simulink model "unitree_a1_bounding"  (R2022b)
settings: Solver=VariableStepAuto  StartTime=0.0  StopTime=10.0  RelTol=1e-3
values from neighbouring files (symbols this model uses):
  m = 12    [mpc.m]    (also in mpc_soln.m; qp_soln.m)
  N = 50    [mpc.m]    (also in mpc_caller.m = params.N; qp_caller.m = params.N)
  X = [p; reshape(R, [9 1]); v; R'*w]    [mpc_caller.m]    (also in qp_caller.m)
undefined symbols (not defined in the file or in its folder): Y, Z
libraries: sm_lib x214, nesl_utility x117, simulink x3
(part 4 of 5)

== system unitree_a1_bounding/Subsystem4 ==
  PS-Simulink Converter : nesl_utility/PS-Simulink Converter  PhysicalDomain=network_engine_domain  SubClassName=ps_output  LeftPortType=input  RightPortType=output  PseudoPeriodic=off  Frequencies=[]  VectorFormat=inherit  Unit=inherit  AffineConversion=off
  PS-Simulink Converter1 : nesl_utility/PS-Simulink Converter  PhysicalDomain=network_engine_domain  SubClassName=ps_output  LeftPortType=input  RightPortType=output  PseudoPeriodic=off  Frequencies=[]  VectorFormat=inherit  Unit=inherit  AffineConversion=off
  PS-Simulink Converter2 : nesl_utility/PS-Simulink Converter  PhysicalDomain=network_engine_domain  SubClassName=ps_output  LeftPortType=input  RightPortType=output  PseudoPeriodic=off  Frequencies=[]  VectorFormat=inherit  Unit=inherit  AffineConversion=off
  1 : PMIOPort  Side=Left
  2 : PMIOPort  Port=2  Side=Left
  3 : PMIOPort  Port=3  Side=Left
  q : Outport
  w : Outport  Port=2
  t : Outport  Port=3
  wires:
  PS-Simulink Converter/1 -> q/1
  PS-Simulink Converter1/1 -> w/1
  PS-Simulink Converter2/1 -> t/1
  connections:
  1/RConn1 -- PS-Simulink Converter/LConn1
  2/RConn1 -- PS-Simulink Converter1/LConn1
  3/RConn1 -- PS-Simulink Converter2/LConn1

== system unitree_a1_bounding/Subsystem5 ==
  PS-Simulink Converter : nesl_utility/PS-Simulink Converter  PhysicalDomain=network_engine_domain  SubClassName=ps_output  LeftPortType=input  RightPortType=output  PseudoPeriodic=off  Frequencies=[]  VectorFormat=inherit  Unit=inherit  AffineConversion=off
  PS-Simulink Converter1 : nesl_utility/PS-Simulink Converter  PhysicalDomain=network_engine_domain  SubClassName=ps_output  LeftPortType=input  RightPortType=output  PseudoPeriodic=off  Frequencies=[]  VectorFormat=inherit  Unit=inherit  AffineConversion=off
  PS-Simulink Converter2 : nesl_utility/PS-Simulink Converter  PhysicalDomain=network_engine_domain  SubClassName=ps_output  LeftPortType=input  RightPortType=output  PseudoPeriodic=off  Frequencies=[]  VectorFormat=inherit  Unit=inherit  AffineConversion=off
  1 : PMIOPort  Side=Left
  2 : PMIOPort  Port=2  Side=Left
  3 : PMIOPort  Port=3  Side=Left
  q : Outport
  w : Outport  Port=2
  t : Outport  Port=3
  wires:
  PS-Simulink Converter/1 -> q/1
  PS-Simulink Converter1/1 -> w/1
  PS-Simulink Converter2/1 -> t/1
  connections:
  1/RConn1 -- PS-Simulink Converter/LConn1
  2/RConn1 -- PS-Simulink Converter1/LConn1
  3/RConn1 -- PS-Simulink Converter2/LConn1

== system unitree_a1_bounding/Subsystem6 ==
  PS-Simulink Converter : nesl_utility/PS-Simulink Converter  PhysicalDomain=network_engine_domain  SubClassName=ps_output  LeftPortType=input  RightPortType=output  PseudoPeriodic=off  Frequencies=[]  VectorFormat=inherit  Unit=inherit  AffineConversion=off
  PS-Simulink Converter1 : nesl_utility/PS-Simulink Converter  PhysicalDomain=network_engine_domain  SubClassName=ps_output  LeftPortType=input  RightPortType=output  PseudoPeriodic=off  Frequencies=[]  VectorFormat=inherit  Unit=inherit  AffineConversion=off
  PS-Simulink Converter2 : nesl_utility/PS-Simulink Converter  PhysicalDomain=network_engine_domain  SubClassName=ps_output  LeftPortType=input  RightPortType=output  PseudoPeriodic=off  Frequencies=[]  VectorFormat=inherit  Unit=inherit  AffineConversion=off
  1 : PMIOPort  Side=Left
  2 : PMIOPort  Port=2  Side=Left
  3 : PMIOPort  Port=3  Side=Left
  q : Outport
  w : Outport  Port=2
  t : Outport  Port=3
  wires:
  PS-Simulink Converter/1 -> q/1
  PS-Simulink Converter1/1 -> w/1
  PS-Simulink Converter2/1 -> t/1
  connections:
  1/RConn1 -- PS-Simulink Converter/LConn1
  2/RConn1 -- PS-Simulink Converter1/LConn1
  3/RConn1 -- PS-Simulink Converter2/LConn1

== system unitree_a1_bounding/Subsystem7 ==
  PS-Simulink Converter : nesl_utility/PS-Simulink Converter  PhysicalDomain=network_engine_domain  SubClassName=ps_output  LeftPortType=input  RightPortType=output  PseudoPeriodic=off  Frequencies=[]  VectorFormat=inherit  Unit=inherit  AffineConversion=off
  PS-Simulink Converter1 : nesl_utility/PS-Simulink Converter  PhysicalDomain=network_engine_domain  SubClassName=ps_output  LeftPortType=input  RightPortType=output  PseudoPeriodic=off  Frequencies=[]  VectorFormat=inherit  Unit=inherit  AffineConversion=off
  PS-Simulink Converter2 : nesl_utility/PS-Simulink Converter  PhysicalDomain=network_engine_domain  SubClassName=ps_output  LeftPortType=input  RightPortType=output  PseudoPeriodic=off  Frequencies=[]  VectorFormat=inherit  Unit=inherit  AffineConversion=off
  1 : PMIOPort  Side=Left
  2 : PMIOPort  Port=2  Side=Left
  3 : PMIOPort  Port=3  Side=Left
  q : Outport
  w : Outport  Port=2
  t : Outport  Port=3
  wires:
  PS-Simulink Converter2/1 -> t/1
  PS-Simulink Converter1/1 -> w/1
  PS-Simulink Converter/1 -> q/1
  connections:
  3/RConn1 -- PS-Simulink Converter2/LConn1
  2/RConn1 -- PS-Simulink Converter1/LConn1
  1/RConn1 -- PS-Simulink Converter/LConn1

== system unitree_a1_bounding/Subsystem8 ==
  PS-Simulink Converter : nesl_utility/PS-Simulink Converter  PhysicalDomain=network_engine_domain  SubClassName=ps_output  LeftPortType=input  RightPortType=output  PseudoPeriodic=off  Frequencies=[]  VectorFormat=inherit  Unit=inherit  AffineConversion=off
  PS-Simulink Converter1 : nesl_utility/PS-Simulink Converter  PhysicalDomain=network_engine_domain  SubClassName=ps_output  LeftPortType=input  RightPortType=output  PseudoPeriodic=off  Frequencies=[]  VectorFormat=inherit  Unit=inherit  AffineConversion=off
  PS-Simulink Converter2 : nesl_utility/PS-Simulink Converter  PhysicalDomain=network_engine_domain  SubClassName=ps_output  LeftPortType=input  RightPortType=output  PseudoPeriodic=off  Frequencies=[]  VectorFormat=inherit  Unit=inherit  AffineConversion=off
  1 : PMIOPort  Side=Left
  2 : PMIOPort  Port=2  Side=Left
  3 : PMIOPort  Port=3  Side=Left
  q : Outport
  w : Outport  Port=2
  t : Outport  Port=3
  wires:
  PS-Simulink Converter2/1 -> t/1
  PS-Simulink Converter1/1 -> w/1
  PS-Simulink Converter/1 -> q/1
  connections:
  3/RConn1 -- PS-Simulink Converter2/LConn1
  2/RConn1 -- PS-Simulink Converter1/LConn1
  1/RConn1 -- PS-Simulink Converter/LConn1

== system unitree_a1_bounding/Subsystem9 ==
  PS-Simulink Converter : nesl_utility/PS-Simulink Converter  PhysicalDomain=network_engine_domain  SubClassName=ps_output  LeftPortType=input  RightPortType=output  PseudoPeriodic=off  Frequencies=[]  VectorFormat=inherit  Unit=inherit  AffineConversion=off
  PS-Simulink Converter1 : nesl_utility/PS-Simulink Converter  PhysicalDomain=network_engine_domain  SubClassName=ps_output  LeftPortType=input  RightPortType=output  PseudoPeriodic=off  Frequencies=[]  VectorFormat=inherit  Unit=inherit  AffineConversion=off
  PS-Simulink Converter2 : nesl_utility/PS-Simulink Converter  PhysicalDomain=network_engine_domain  SubClassName=ps_output  LeftPortType=input  RightPortType=output  PseudoPeriodic=off  Frequencies=[]  VectorFormat=inherit  Unit=inherit  AffineConversion=off
  1 : PMIOPort  Side=Left
  2 : PMIOPort  Port=2  Side=Left
  3 : PMIOPort  Port=3  Side=Left
  q : Outport
  w : Outport  Port=2
  t : Outport  Port=3
  wires:
  PS-Simulink Converter2/1 -> t/1
  PS-Simulink Converter1/1 -> w/1
  PS-Simulink Converter/1 -> q/1
  connections:
  3/RConn1 -- PS-Simulink Converter2/LConn1
  2/RConn1 -- PS-Simulink Converter1/LConn1
  1/RConn1 -- PS-Simulink Converter/LConn1

== system unitree_a1_bounding/base ==
  ReferenceFrame : sm_lib/Frames and Transforms/Reference Frame
  Visual : sm_lib/Body Elements/Brick Solid  GraphicAmbientColor=[0.15 0.15 0.15 1.0]  BasedOnType=Density  BrickDimensions=[0.001, 0.001, 0.001]  BrickDimensionUnits=m  CenterOfMass=[0, 0, 0]  CenterOfMassUnits=m  GraphicDiffuseColor=[0.5, 0.5, 0.5]  Density=1000  DensityUnits=kg/m^3  DoExposeReferenceFrame=on  GraphicEmissiveColor=[0.0 0.0 0.0 1.0]  ExportEntireGeometry=off  SerializedFrames=<Frames/>  MarkerShape=Sphere  MarkerSize=10  GraphicType=FromGeometry  InertiaType=Custom  Mass=0  MassUnits=kg  MomentsOfInertia=[0, 0, 0]  MomentsOfInertiaUnits=kg*m^2  GraphicOpacity=1  ProductsOfInertia=[0, 0, 0]  ProductsOfInertiaUnits=kg*m^2  GraphicShininess=75  GraphicSpecularColor=[0.5 0.5 0.5 1.0]  GraphicVisPropType=SimpleVisualProperties
  VisualOriginTransform : sm_lib/Frames and Transforms/Rigid Transform  TranslationMethod=Cartesian  TranslationStandardOffset=0  TranslationLengthUnit=m  TranslationStandardAxis=+Z  TranslationCartesianOffset=[0, 0, 0]  TranslationROffset=0  TranslationROffsetUnits=m  TranslationZOffset=0  TranslationZOffsetUnits=m  TranslationThetaOffset=0  TranslationThetaOffsetUnits=deg  RotationMethod=RotationSequence  RotationAngleUnits=deg  RotationStandardAxis=+Z  RotationAngle=0.0  RotationArbitraryAxis=[0 0 1]  FollAlignAxisA=+X  BaseAlignAxisA=+Y  FollAlignAxisB=+Y  BaseAlignAxisB=+Z  RotationSequenceAxes=BaseAxes  RotationSequence=XYZ  RotationSequenceAngles=[0, 0, 0]  RotationSequenceAnglesUnits=rad  RotationMatrix=[1 0 0; 0 1 0; 0 0 1]  Quaternion=[1 0 0 0]
  floating_base_OriginTransform : sm_lib/Frames and Transforms/Rigid Transform  TranslationMethod=Cartesian  TranslationStandardOffset=0  TranslationLengthUnit=m  TranslationStandardAxis=+Z  TranslationCartesianOffset=[0, 0, 0]  TranslationROffset=0  TranslationROffsetUnits=m  TranslationZOffset=0  TranslationZOffsetUnits=m  TranslationThetaOffset=0  TranslationThetaOffsetUnits=deg  RotationMethod=RotationSequence  RotationAngleUnits=deg  RotationStandardAxis=+Z  RotationAngle=0.0  RotationArbitraryAxis=[0 0 1]  FollAlignAxisA=+X  BaseAlignAxisA=+Y  FollAlignAxisB=+Y  BaseAlignAxisB=+Z  RotationSequenceAxes=BaseAxes  RotationSequence=XYZ  RotationSequenceAngles=[0, 0, 0]  RotationSequenceAnglesUnits=rad  RotationMatrix=[1 0 0; 0 1 0; 0 0 1]  Quaternion=[1 0 0 0]
  F : PMIOPort  Side=Left
  F1 : PMIOPort  Port=2  Side=Right
  connections:
  VisualOriginTransform/LConn1 -- ReferenceFrame/RConn1 -- F/RConn1 -- floating_base_OriginTransform/LConn1
  Visual/RConn1 -- VisualOriginTransform/RConn1
  floating_base_OriginTransform/RConn1 -- F1/RConn1

== system unitree_a1_bounding/imu_link ==
  Inertia : sm_lib/Body Elements/Inertia  InertiaType=Custom  Mass=0.001  MassUnits=kg  CenterOfMass=[0, 0, 0]  CenterOfMassUnits=m  MomentsOfInertia=[0.0001, 0.0001, 0.0001]  MomentsOfInertiaUnits=kg*m^2  ProductsOfInertia=[0, 0, 0]  ProductsOfInertiaUnits=kg*m^2  GraphicType=None  MarkerShape=Inertia  MarkerSize=20  GraphicVisPropType=SimpleVisualProperties  GraphicDiffuseColor=[0.5 0.5 0.5]  GraphicSpecularColor=[0.5 0.5 0.5 1.0]  GraphicAmbientColor=[0.15 0.15 0.15 1.0]  GraphicEmissiveColor=[0.0 0.0 0.0 1.0]  GraphicShininess=75  GraphicOpacity=1.0
  InertiaOriginTransform : sm_lib/Frames and Transforms/Rigid Transform  TranslationMethod=Cartesian  TranslationStandardOffset=0  TranslationLengthUnit=m  TranslationStandardAxis=+Z  TranslationCartesianOffset=[0, 0, 0]  TranslationROffset=0  TranslationROffsetUnits=m  TranslationZOffset=0  TranslationZOffsetUnits=m  TranslationThetaOffset=0  TranslationThetaOffsetUnits=deg  RotationMethod=RotationSequence  RotationAngleUnits=deg  RotationStandardAxis=+Z  RotationAngle=0.0  RotationArbitraryAxis=[0 0 1]  FollAlignAxisA=+X  BaseAlignAxisA=+Y  FollAlignAxisB=+Y  BaseAlignAxisB=+Z  RotationSequenceAxes=BaseAxes  RotationSequence=XYZ  RotationSequenceAngles=[0, 0, 0]  RotationSequenceAnglesUnits=rad  RotationMatrix=[1 0 0; 0 1 0; 0 0 1]  Quaternion=[1 0 0 0]
  ReferenceFrame : sm_lib/Frames and Transforms/Reference Frame
  Visual : sm_lib/Body Elements/Brick Solid  GraphicAmbientColor=[0.15 0.15 0.15 1.0]  BasedOnType=Density  BrickDimensions=[0.001, 0.001, 0.001]  BrickDimensionUnits=m  CenterOfMass=[0, 0, 0]  CenterOfMassUnits=m  GraphicDiffuseColor=[0.8, 0, 0]  Density=1000  DensityUnits=kg/m^3  DoExposeReferenceFrame=on  GraphicEmissiveColor=[0.0 0.0 0.0 1.0]  ExportEntireGeometry=off  SerializedFrames=<Frames/>  MarkerShape=Sphere  MarkerSize=10  GraphicType=FromGeometry  InertiaType=Custom  Mass=0  MassUnits=kg  MomentsOfInertia=[0, 0, 0]  MomentsOfInertiaUnits=kg*m^2  GraphicOpacity=1  ProductsOfInertia=[0, 0, 0]  ProductsOfInertiaUnits=kg*m^2  GraphicShininess=75  GraphicSpecularColor=[0.5 0.5 0.5 1.0]  GraphicVisPropType=SimpleVisualProperties
  VisualOriginTransform : sm_lib/Frames and Transforms/Rigid Transform  TranslationMethod=Cartesian  TranslationStandardOffset=0  TranslationLengthUnit=m  TranslationStandardAxis=+Z  TranslationCartesianOffset=[0, 0, 0]  TranslationROffset=0  TranslationROffsetUnits=m  TranslationZOffset=0  TranslationZOffsetUnits=m  TranslationThetaOffset=0  TranslationThetaOffsetUnits=deg  RotationMethod=RotationSequence  RotationAngleUnits=deg  RotationStandardAxis=+Z  RotationAngle=0.0  RotationArbitraryAxis=[0 0 1]  FollAlignAxisA=+X  BaseAlignAxisA=+Y  FollAlignAxisB=+Y  BaseAlignAxisB=+Z  RotationSequenceAxes=BaseAxes  RotationSequence=XYZ  RotationSequenceAngles=[0, 0, 0]  RotationSequenceAnglesUnits=rad  RotationMatrix=[1 0 0; 0 1 0; 0 0 1]  Quaternion=[1 0 0 0]
  F : PMIOPort  Side=Left
  connections:
  Inertia/RConn1 -- InertiaOriginTransform/RConn1
  ReferenceFrame/RConn1 -- InertiaOriginTransform/LConn1 -- VisualOriginTransform/LConn1 -- F/RConn1
  Visual/RConn1 -- VisualOriginTransform/RConn1

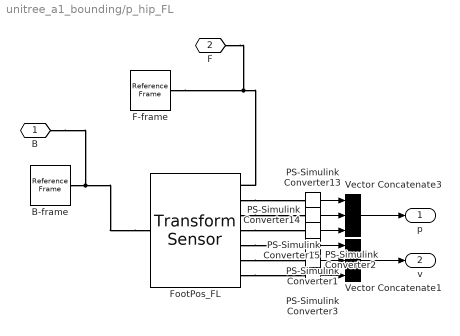
== system unitree_a1_bounding/p_hip_FL ==
  B-frame : sm_lib/Frames and Transforms/Reference Frame
  F-frame : sm_lib/Frames and Transforms/Reference Frame
  FootPos_FL : sm_lib/Frames and Transforms/Transform Sensor  MeasurementFrame=World  SenseAngle=off  SenseAxis=off  SenseQ=off  SenseR=off  SenseRotationSequence=off  RotationSequence=XYX  SenseOmegaX=off  SenseOmegaY=off  SenseOmegaZ=off  SenseQDot=off  SenseRDot=off  SenseAlphaX=off  SenseAlphaY=off  SenseAlphaZ=off  SenseQDDot=off  SenseRDDot=off  SenseX=on  SenseY=on  SenseZ=on  SenseRad=off  SenseAzim=off  SenseDist=off  SenseInc=off  SenseXDot=on  SenseYDot=on  SenseZDot=on  SenseRadDot=off  SenseAzimDot=off  SenseDistDot=off  SenseIncDot=off  SenseXDDot=off  SenseYDDot=off  SenseZDDot=off  SenseRadDDot=off  SenseAzimDDot=off  SenseDistDDot=off  SenseIncDDot=off
  PS-Simulink Converter{1..3,13..15} (6 alike) : nesl_utility/PS-Simulink Converter  PhysicalDomain=network_engine_domain  SubClassName=ps_output  LeftPortType=input  RightPortType=output  PseudoPeriodic=off  Frequencies=[]  VectorFormat=inherit  Unit=inherit  AffineConversion=off
  Vector Concatenate1 : Concatenate  NumInputs=3
  Vector Concatenate3 : Concatenate  NumInputs=3
  B : PMIOPort  Side=Left
  F : PMIOPort  Port=2  Side=Left
  p : Outport
  v : Outport  Port=2
  wires:
  PS-Simulink Converter13/1 -> Vector Concatenate3/1
  PS-Simulink Converter15/1 -> Vector Concatenate3/3
  PS-Simulink Converter14/1 -> Vector Concatenate3/2
  Vector Concatenate3/1 -> p/1
  PS-Simulink Converter2/1 -> Vector Concatenate1/2
  PS-Simulink Converter3/1 -> Vector Concatenate1/3
  PS-Simulink Converter1/1 -> Vector Concatenate1/1
  Vector Concatenate1/1 -> v/1
  connections:
  FootPos_FL/LConn1 -- B-frame/RConn1 -- B/RConn1
  FootPos_FL/RConn1 -- F-frame/RConn1 -- F/RConn1
  FootPos_FL/RConn4 -- PS-Simulink Converter15/LConn1
  FootPos_FL/RConn2 -- PS-Simulink Converter13/LConn1
  FootPos_FL/RConn3 -- PS-Simulink Converter14/LConn1
  FootPos_FL/RConn6 -- PS-Simulink Converter2/LConn1
  FootPos_FL/RConn5 -- PS-Simulink Converter1/LConn1
  FootPos_FL/RConn7 -- PS-Simulink Converter3/LConn1

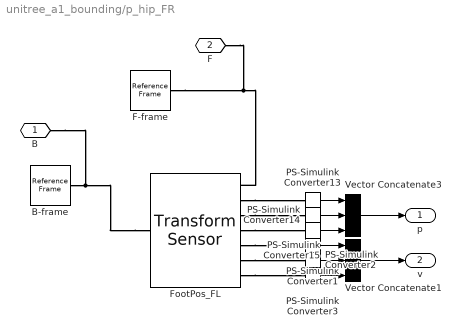
== system unitree_a1_bounding/p_hip_FR ==
  B-frame : sm_lib/Frames and Transforms/Reference Frame
  F-frame : sm_lib/Frames and Transforms/Reference Frame
  FootPos_FL : sm_lib/Frames and Transforms/Transform Sensor  MeasurementFrame=World  SenseAngle=off  SenseAxis=off  SenseQ=off  SenseR=off  SenseRotationSequence=off  RotationSequence=XYX  SenseOmegaX=off  SenseOmegaY=off  SenseOmegaZ=off  SenseQDot=off  SenseRDot=off  SenseAlphaX=off  SenseAlphaY=off  SenseAlphaZ=off  SenseQDDot=off  SenseRDDot=off  SenseX=on  SenseY=on  SenseZ=on  SenseRad=off  SenseAzim=off  SenseDist=off  SenseInc=off  SenseXDot=on  SenseYDot=on  SenseZDot=on  SenseRadDot=off  SenseAzimDot=off  SenseDistDot=off  SenseIncDot=off  SenseXDDot=off  SenseYDDot=off  SenseZDDot=off  SenseRadDDot=off  SenseAzimDDot=off  SenseDistDDot=off  SenseIncDDot=off
  PS-Simulink Converter{1..3,13..15} (6 alike) : nesl_utility/PS-Simulink Converter  PhysicalDomain=network_engine_domain  SubClassName=ps_output  LeftPortType=input  RightPortType=output  PseudoPeriodic=off  Frequencies=[]  VectorFormat=inherit  Unit=inherit  AffineConversion=off
  Vector Concatenate1 : Concatenate  NumInputs=3
  Vector Concatenate3 : Concatenate  NumInputs=3
  B : PMIOPort  Side=Left
  F : PMIOPort  Port=2  Side=Left
  p : Outport
  v : Outport  Port=2
  wires:
  PS-Simulink Converter13/1 -> Vector Concatenate3/1
  PS-Simulink Converter15/1 -> Vector Concatenate3/3
  PS-Simulink Converter14/1 -> Vector Concatenate3/2
  Vector Concatenate3/1 -> p/1
  PS-Simulink Converter2/1 -> Vector Concatenate1/2
  PS-Simulink Converter3/1 -> Vector Concatenate1/3
  PS-Simulink Converter1/1 -> Vector Concatenate1/1
  Vector Concatenate1/1 -> v/1
  connections:
  FootPos_FL/LConn1 -- B-frame/RConn1 -- B/RConn1
  FootPos_FL/RConn1 -- F-frame/RConn1 -- F/RConn1
  FootPos_FL/RConn4 -- PS-Simulink Converter15/LConn1
  FootPos_FL/RConn2 -- PS-Simulink Converter13/LConn1
  FootPos_FL/RConn3 -- PS-Simulink Converter14/LConn1
  FootPos_FL/RConn6 -- PS-Simulink Converter2/LConn1
  FootPos_FL/RConn5 -- PS-Simulink Converter1/LConn1
  FootPos_FL/RConn7 -- PS-Simulink Converter3/LConn1

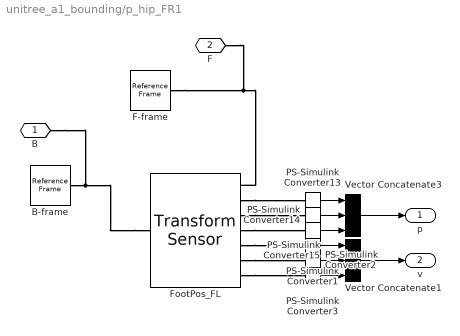
== system unitree_a1_bounding/p_hip_FR1 ==
  B-frame : sm_lib/Frames and Transforms/Reference Frame
  F-frame : sm_lib/Frames and Transforms/Reference Frame
  FootPos_FL : sm_lib/Frames and Transforms/Transform Sensor  MeasurementFrame=World  SenseAngle=off  SenseAxis=off  SenseQ=off  SenseR=off  SenseRotationSequence=off  RotationSequence=XYX  SenseOmegaX=off  SenseOmegaY=off  SenseOmegaZ=off  SenseQDot=off  SenseRDot=off  SenseAlphaX=off  SenseAlphaY=off  SenseAlphaZ=off  SenseQDDot=off  SenseRDDot=off  SenseX=on  SenseY=on  SenseZ=on  SenseRad=off  SenseAzim=off  SenseDist=off  SenseInc=off  SenseXDot=on  SenseYDot=on  SenseZDot=on  SenseRadDot=off  SenseAzimDot=off  SenseDistDot=off  SenseIncDot=off  SenseXDDot=off  SenseYDDot=off  SenseZDDot=off  SenseRadDDot=off  SenseAzimDDot=off  SenseDistDDot=off  SenseIncDDot=off
  PS-Simulink Converter{1..3,13..15} (6 alike) : nesl_utility/PS-Simulink Converter  PhysicalDomain=network_engine_domain  SubClassName=ps_output  LeftPortType=input  RightPortType=output  PseudoPeriodic=off  Frequencies=[]  VectorFormat=inherit  Unit=inherit  AffineConversion=off
  Vector Concatenate1 : Concatenate  NumInputs=3
  Vector Concatenate3 : Concatenate  NumInputs=3
  B : PMIOPort  Side=Left
  F : PMIOPort  Port=2  Side=Left
  p : Outport
  v : Outport  Port=2
  wires:
  PS-Simulink Converter13/1 -> Vector Concatenate3/1
  PS-Simulink Converter15/1 -> Vector Concatenate3/3
  PS-Simulink Converter14/1 -> Vector Concatenate3/2
  Vector Concatenate3/1 -> p/1
  PS-Simulink Converter2/1 -> Vector Concatenate1/2
  PS-Simulink Converter3/1 -> Vector Concatenate1/3
  PS-Simulink Converter1/1 -> Vector Concatenate1/1
  Vector Concatenate1/1 -> v/1
  connections:
  FootPos_FL/LConn1 -- B-frame/RConn1 -- B/RConn1
  FootPos_FL/RConn1 -- F-frame/RConn1 -- F/RConn1
  FootPos_FL/RConn4 -- PS-Simulink Converter15/LConn1
  FootPos_FL/RConn2 -- PS-Simulink Converter13/LConn1
  FootPos_FL/RConn3 -- PS-Simulink Converter14/LConn1
  FootPos_FL/RConn6 -- PS-Simulink Converter2/LConn1
  FootPos_FL/RConn5 -- PS-Simulink Converter1/LConn1
  FootPos_FL/RConn7 -- PS-Simulink Converter3/LConn1

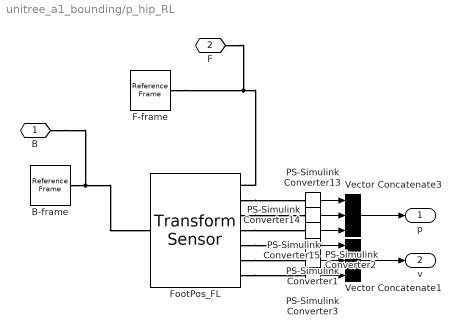
== system unitree_a1_bounding/p_hip_RL ==
  B-frame : sm_lib/Frames and Transforms/Reference Frame
  F-frame : sm_lib/Frames and Transforms/Reference Frame
  FootPos_FL : sm_lib/Frames and Transforms/Transform Sensor  MeasurementFrame=World  SenseAngle=off  SenseAxis=off  SenseQ=off  SenseR=off  SenseRotationSequence=off  RotationSequence=XYX  SenseOmegaX=off  SenseOmegaY=off  SenseOmegaZ=off  SenseQDot=off  SenseRDot=off  SenseAlphaX=off  SenseAlphaY=off  SenseAlphaZ=off  SenseQDDot=off  SenseRDDot=off  SenseX=on  SenseY=on  SenseZ=on  SenseRad=off  SenseAzim=off  SenseDist=off  SenseInc=off  SenseXDot=on  SenseYDot=on  SenseZDot=on  SenseRadDot=off  SenseAzimDot=off  SenseDistDot=off  SenseIncDot=off  SenseXDDot=off  SenseYDDot=off  SenseZDDot=off  SenseRadDDot=off  SenseAzimDDot=off  SenseDistDDot=off  SenseIncDDot=off
  PS-Simulink Converter{1..3,13..15} (6 alike) : nesl_utility/PS-Simulink Converter  PhysicalDomain=network_engine_domain  SubClassName=ps_output  LeftPortType=input  RightPortType=output  PseudoPeriodic=off  Frequencies=[]  VectorFormat=inherit  Unit=inherit  AffineConversion=off
  Vector Concatenate1 : Concatenate  NumInputs=3
  Vector Concatenate3 : Concatenate  NumInputs=3
  B : PMIOPort  Side=Left
  F : PMIOPort  Port=2  Side=Left
  p : Outport
  v : Outport  Port=2
  wires:
  Vector Concatenate1/1 -> v/1
  PS-Simulink Converter1/1 -> Vector Concatenate1/1
  PS-Simulink Converter3/1 -> Vector Concatenate1/3
  PS-Simulink Converter2/1 -> Vector Concatenate1/2
  Vector Concatenate3/1 -> p/1
  PS-Simulink Converter14/1 -> Vector Concatenate3/2
  PS-Simulink Converter15/1 -> Vector Concatenate3/3
  PS-Simulink Converter13/1 -> Vector Concatenate3/1
  connections:
  FootPos_FL/RConn7 -- PS-Simulink Converter3/LConn1
  FootPos_FL/RConn5 -- PS-Simulink Converter1/LConn1
  FootPos_FL/RConn6 -- PS-Simulink Converter2/LConn1
  FootPos_FL/RConn3 -- PS-Simulink Converter14/LConn1
  FootPos_FL/RConn2 -- PS-Simulink Converter13/LConn1
  FootPos_FL/RConn4 -- PS-Simulink Converter15/LConn1
  F/RConn1 -- F-frame/RConn1 -- FootPos_FL/RConn1
  B/RConn1 -- B-frame/RConn1 -- FootPos_FL/LConn1

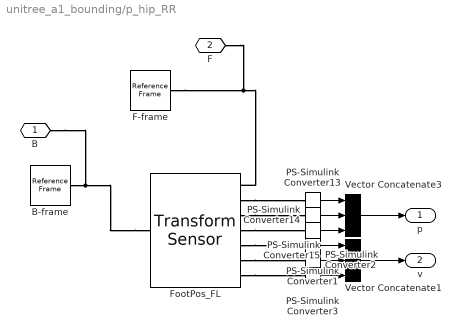
== system unitree_a1_bounding/p_hip_RR ==
  B-frame : sm_lib/Frames and Transforms/Reference Frame
  F-frame : sm_lib/Frames and Transforms/Reference Frame
  FootPos_FL : sm_lib/Frames and Transforms/Transform Sensor  MeasurementFrame=World  SenseAngle=off  SenseAxis=off  SenseQ=off  SenseR=off  SenseRotationSequence=off  RotationSequence=XYX  SenseOmegaX=off  SenseOmegaY=off  SenseOmegaZ=off  SenseQDot=off  SenseRDot=off  SenseAlphaX=off  SenseAlphaY=off  SenseAlphaZ=off  SenseQDDot=off  SenseRDDot=off  SenseX=on  SenseY=on  SenseZ=on  SenseRad=off  SenseAzim=off  SenseDist=off  SenseInc=off  SenseXDot=on  SenseYDot=on  SenseZDot=on  SenseRadDot=off  SenseAzimDot=off  SenseDistDot=off  SenseIncDot=off  SenseXDDot=off  SenseYDDot=off  SenseZDDot=off  SenseRadDDot=off  SenseAzimDDot=off  SenseDistDDot=off  SenseIncDDot=off
  PS-Simulink Converter{1..3,13..15} (6 alike) : nesl_utility/PS-Simulink Converter  PhysicalDomain=network_engine_domain  SubClassName=ps_output  LeftPortType=input  RightPortType=output  PseudoPeriodic=off  Frequencies=[]  VectorFormat=inherit  Unit=inherit  AffineConversion=off
  Vector Concatenate1 : Concatenate  NumInputs=3
  Vector Concatenate3 : Concatenate  NumInputs=3
  B : PMIOPort  Side=Left
  F : PMIOPort  Port=2  Side=Left
  p : Outport
  v : Outport  Port=2
  wires:
  PS-Simulink Converter13/1 -> Vector Concatenate3/1
  PS-Simulink Converter15/1 -> Vector Concatenate3/3
  PS-Simulink Converter14/1 -> Vector Concatenate3/2
  Vector Concatenate3/1 -> p/1
  PS-Simulink Converter2/1 -> Vector Concatenate1/2
  PS-Simulink Converter3/1 -> Vector Concatenate1/3
  PS-Simulink Converter1/1 -> Vector Concatenate1/1
  Vector Concatenate1/1 -> v/1
  connections:
  FootPos_FL/LConn1 -- B-frame/RConn1 -- B/RConn1
  FootPos_FL/RConn1 -- F-frame/RConn1 -- F/RConn1
  FootPos_FL/RConn4 -- PS-Simulink Converter15/LConn1
  FootPos_FL/RConn2 -- PS-Simulink Converter13/LConn1
  FootPos_FL/RConn3 -- PS-Simulink Converter14/LConn1
  FootPos_FL/RConn6 -- PS-Simulink Converter2/LConn1
  FootPos_FL/RConn5 -- PS-Simulink Converter1/LConn1
  FootPos_FL/RConn7 -- PS-Simulink Converter3/LConn1

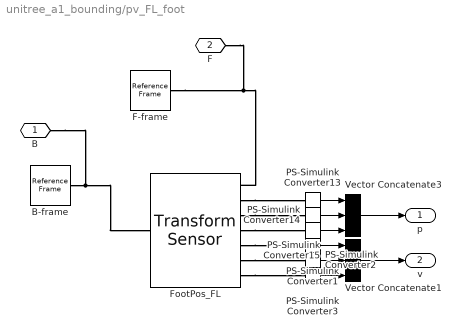
== system unitree_a1_bounding/pv_FL_foot ==
  B-frame : sm_lib/Frames and Transforms/Reference Frame
  F-frame : sm_lib/Frames and Transforms/Reference Frame
  FootPos_FL : sm_lib/Frames and Transforms/Transform Sensor  MeasurementFrame=World  SenseAngle=off  SenseAxis=off  SenseQ=off  SenseR=off  SenseRotationSequence=off  RotationSequence=XYX  SenseOmegaX=off  SenseOmegaY=off  SenseOmegaZ=off  SenseQDot=off  SenseRDot=off  SenseAlphaX=off  SenseAlphaY=off  SenseAlphaZ=off  SenseQDDot=off  SenseRDDot=off  SenseX=on  SenseY=on  SenseZ=on  SenseRad=off  SenseAzim=off  SenseDist=off  SenseInc=off  SenseXDot=on  SenseYDot=on  SenseZDot=on  SenseRadDot=off  SenseAzimDot=off  SenseDistDot=off  SenseIncDot=off  SenseXDDot=off  SenseYDDot=off  SenseZDDot=off  SenseRadDDot=off  SenseAzimDDot=off  SenseDistDDot=off  SenseIncDDot=off
  PS-Simulink Converter{1..3,13..15} (6 alike) : nesl_utility/PS-Simulink Converter  PhysicalDomain=network_engine_domain  SubClassName=ps_output  LeftPortType=input  RightPortType=output  PseudoPeriodic=off  Frequencies=[]  VectorFormat=inherit  Unit=inherit  AffineConversion=off
  Vector Concatenate1 : Concatenate  NumInputs=3
  Vector Concatenate3 : Concatenate  NumInputs=3
  B : PMIOPort  Side=Left
  F : PMIOPort  Port=2  Side=Left
  p : Outport
  v : Outport  Port=2
  wires:
  PS-Simulink Converter13/1 -> Vector Concatenate3/1
  PS-Simulink Converter15/1 -> Vector Concatenate3/3
  PS-Simulink Converter14/1 -> Vector Concatenate3/2
  Vector Concatenate3/1 -> p/1
  PS-Simulink Converter2/1 -> Vector Concatenate1/2
  PS-Simulink Converter3/1 -> Vector Concatenate1/3
  PS-Simulink Converter1/1 -> Vector Concatenate1/1
  Vector Concatenate1/1 -> v/1
  connections:
  B-frame/RConn1 -- B/RConn1 -- FootPos_FL/LConn1
  F-frame/RConn1 -- F/RConn1 -- FootPos_FL/RConn1
  FootPos_FL/RConn4 -- PS-Simulink Converter15/LConn1
  FootPos_FL/RConn2 -- PS-Simulink Converter13/LConn1
  FootPos_FL/RConn3 -- PS-Simulink Converter14/LConn1
  FootPos_FL/RConn6 -- PS-Simulink Converter2/LConn1
  FootPos_FL/RConn5 -- PS-Simulink Converter1/LConn1
  FootPos_FL/RConn7 -- PS-Simulink Converter3/LConn1

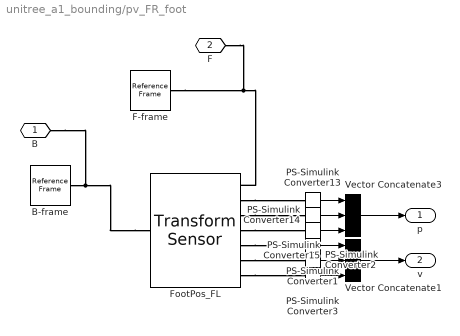
== system unitree_a1_bounding/pv_FR_foot ==
  B-frame : sm_lib/Frames and Transforms/Reference Frame
  F-frame : sm_lib/Frames and Transforms/Reference Frame
  FootPos_FL : sm_lib/Frames and Transforms/Transform Sensor  MeasurementFrame=World  SenseAngle=off  SenseAxis=off  SenseQ=off  SenseR=off  SenseRotationSequence=off  RotationSequence=XYX  SenseOmegaX=off  SenseOmegaY=off  SenseOmegaZ=off  SenseQDot=off  SenseRDot=off  SenseAlphaX=off  SenseAlphaY=off  SenseAlphaZ=off  SenseQDDot=off  SenseRDDot=off  SenseX=on  SenseY=on  SenseZ=on  SenseRad=off  SenseAzim=off  SenseDist=off  SenseInc=off  SenseXDot=on  SenseYDot=on  SenseZDot=on  SenseRadDot=off  SenseAzimDot=off  SenseDistDot=off  SenseIncDot=off  SenseXDDot=off  SenseYDDot=off  SenseZDDot=off  SenseRadDDot=off  SenseAzimDDot=off  SenseDistDDot=off  SenseIncDDot=off
  PS-Simulink Converter{1..3,13..15} (6 alike) : nesl_utility/PS-Simulink Converter  PhysicalDomain=network_engine_domain  SubClassName=ps_output  LeftPortType=input  RightPortType=output  PseudoPeriodic=off  Frequencies=[]  VectorFormat=inherit  Unit=inherit  AffineConversion=off
  Vector Concatenate1 : Concatenate  NumInputs=3
  Vector Concatenate3 : Concatenate  NumInputs=3
  B : PMIOPort  Side=Left
  F : PMIOPort  Port=2  Side=Left
  p : Outport
  v : Outport  Port=2
  wires:
  PS-Simulink Converter13/1 -> Vector Concatenate3/1
  PS-Simulink Converter15/1 -> Vector Concatenate3/3
  PS-Simulink Converter14/1 -> Vector Concatenate3/2
  Vector Concatenate3/1 -> p/1
  PS-Simulink Converter2/1 -> Vector Concatenate1/2
  PS-Simulink Converter3/1 -> Vector Concatenate1/3
  PS-Simulink Converter1/1 -> Vector Concatenate1/1
  Vector Concatenate1/1 -> v/1
  connections:
  FootPos_FL/LConn1 -- B-frame/RConn1 -- B/RConn1
  FootPos_FL/RConn1 -- F-frame/RConn1 -- F/RConn1
  FootPos_FL/RConn4 -- PS-Simulink Converter15/LConn1
  FootPos_FL/RConn2 -- PS-Simulink Converter13/LConn1
  FootPos_FL/RConn3 -- PS-Simulink Converter14/LConn1
  FootPos_FL/RConn6 -- PS-Simulink Converter2/LConn1
  FootPos_FL/RConn5 -- PS-Simulink Converter1/LConn1
  FootPos_FL/RConn7 -- PS-Simulink Converter3/LConn1

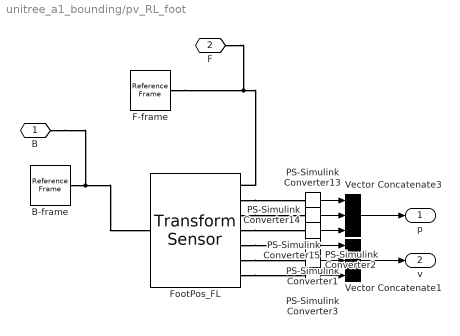
== system unitree_a1_bounding/pv_RL_foot ==
  B-frame : sm_lib/Frames and Transforms/Reference Frame
  F-frame : sm_lib/Frames and Transforms/Reference Frame
  FootPos_FL : sm_lib/Frames and Transforms/Transform Sensor  MeasurementFrame=World  SenseAngle=off  SenseAxis=off  SenseQ=off  SenseR=off  SenseRotationSequence=off  RotationSequence=XYX  SenseOmegaX=off  SenseOmegaY=off  SenseOmegaZ=off  SenseQDot=off  SenseRDot=off  SenseAlphaX=off  SenseAlphaY=off  SenseAlphaZ=off  SenseQDDot=off  SenseRDDot=off  SenseX=on  SenseY=on  SenseZ=on  SenseRad=off  SenseAzim=off  SenseDist=off  SenseInc=off  SenseXDot=on  SenseYDot=on  SenseZDot=on  SenseRadDot=off  SenseAzimDot=off  SenseDistDot=off  SenseIncDot=off  SenseXDDot=off  SenseYDDot=off  SenseZDDot=off  SenseRadDDot=off  SenseAzimDDot=off  SenseDistDDot=off  SenseIncDDot=off
  PS-Simulink Converter{1..3,13..15} (6 alike) : nesl_utility/PS-Simulink Converter  PhysicalDomain=network_engine_domain  SubClassName=ps_output  LeftPortType=input  RightPortType=output  PseudoPeriodic=off  Frequencies=[]  VectorFormat=inherit  Unit=inherit  AffineConversion=off
  Vector Concatenate1 : Concatenate  NumInputs=3
  Vector Concatenate3 : Concatenate  NumInputs=3
  B : PMIOPort  Side=Left
  F : PMIOPort  Port=2  Side=Left
  p : Outport
  v : Outport  Port=2
  wires:
  Vector Concatenate1/1 -> v/1
  PS-Simulink Converter1/1 -> Vector Concatenate1/1
  PS-Simulink Converter3/1 -> Vector Concatenate1/3
  PS-Simulink Converter2/1 -> Vector Concatenate1/2
  Vector Concatenate3/1 -> p/1
  PS-Simulink Converter14/1 -> Vector Concatenate3/2
  PS-Simulink Converter15/1 -> Vector Concatenate3/3
  PS-Simulink Converter13/1 -> Vector Concatenate3/1
  connections:
  FootPos_FL/RConn7 -- PS-Simulink Converter3/LConn1
  FootPos_FL/RConn5 -- PS-Simulink Converter1/LConn1
  FootPos_FL/RConn6 -- PS-Simulink Converter2/LConn1
  FootPos_FL/RConn3 -- PS-Simulink Converter14/LConn1
  FootPos_FL/RConn2 -- PS-Simulink Converter13/LConn1
  FootPos_FL/RConn4 -- PS-Simulink Converter15/LConn1
  F/RConn1 -- F-frame/RConn1 -- FootPos_FL/RConn1
  B/RConn1 -- B-frame/RConn1 -- FootPos_FL/LConn1

== system unitree_a1_bounding/pv_RR_foot ==
  B-frame : sm_lib/Frames and Transforms/Reference Frame
  F-frame : sm_lib/Frames and Transforms/Reference Frame
  FootPos_FL : sm_lib/Frames and Transforms/Transform Sensor  MeasurementFrame=World  SenseAngle=off  SenseAxis=off  SenseQ=off  SenseR=off  SenseRotationSequence=off  RotationSequence=XYX  SenseOmegaX=off  SenseOmegaY=off  SenseOmegaZ=off  SenseQDot=off  SenseRDot=off  SenseAlphaX=off  SenseAlphaY=off  SenseAlphaZ=off  SenseQDDot=off  SenseRDDot=off  SenseX=on  SenseY=on  SenseZ=on  SenseRad=off  SenseAzim=off  SenseDist=off  SenseInc=off  SenseXDot=on  SenseYDot=on  SenseZDot=on  SenseRadDot=off  SenseAzimDot=off  SenseDistDot=off  SenseIncDot=off  SenseXDDot=off  SenseYDDot=off  SenseZDDot=off  SenseRadDDot=off  SenseAzimDDot=off  SenseDistDDot=off  SenseIncDDot=off
  PS-Simulink Converter{1..3,13..15} (6 alike) : nesl_utility/PS-Simulink Converter  PhysicalDomain=network_engine_domain  SubClassName=ps_output  LeftPortType=input  RightPortType=output  PseudoPeriodic=off  Frequencies=[]  VectorFormat=inherit  Unit=inherit  AffineConversion=off
  Vector Concatenate1 : Concatenate  NumInputs=3
  Vector Concatenate3 : Concatenate  NumInputs=3
  B : PMIOPort  Side=Left
  F : PMIOPort  Port=2  Side=Left
  p : Outport
  v : Outport  Port=2
  wires:
  PS-Simulink Converter13/1 -> Vector Concatenate3/1
  PS-Simulink Converter15/1 -> Vector Concatenate3/3
  PS-Simulink Converter14/1 -> Vector Concatenate3/2
  Vector Concatenate3/1 -> p/1
  PS-Simulink Converter2/1 -> Vector Concatenate1/2
  PS-Simulink Converter3/1 -> Vector Concatenate1/3
  PS-Simulink Converter1/1 -> Vector Concatenate1/1
  Vector Concatenate1/1 -> v/1
  connections:
  FootPos_FL/LConn1 -- B-frame/RConn1 -- B/RConn1
  FootPos_FL/RConn1 -- F-frame/RConn1 -- F/RConn1
  FootPos_FL/RConn4 -- PS-Simulink Converter15/LConn1
  FootPos_FL/RConn2 -- PS-Simulink Converter13/LConn1
  FootPos_FL/RConn3 -- PS-Simulink Converter14/LConn1
  FootPos_FL/RConn6 -- PS-Simulink Converter2/LConn1
  FootPos_FL/RConn5 -- PS-Simulink Converter1/LConn1
  FootPos_FL/RConn7 -- PS-Simulink Converter3/LConn1

== system unitree_a1_bounding/q ==
  RR_calf : Inport
  RL_calf : Inport  Port=2
  FR_calf : Inport  Port=3
  FL_calf : Inport  Port=4
  RR_thigh : Inport  Port=5
  RL_thigh : Inport  Port=6
  FR_thigh : Inport  Port=7
  FL_thigh : Inport  Port=8
  RR_hip : Inport  Port=9
  RL_hip : Inport  Port=10
  FR_hip : Inport  Port=11
  FL_hip : Inport  Port=12
  Joint Angles : Scope  NumInputPorts=12
  Vector Concatenate : Concatenate  NumInputs=12
  joint vector : Outport
  wires:
  RR_calf/1 -> Joint Angles/1, Vector Concatenate/1
  RL_calf/1 -> Joint Angles/2, Vector Concatenate/2
  FR_calf/1 -> Joint Angles/3, Vector Concatenate/3
  FL_calf/1 -> Joint Angles/4, Vector Concatenate/4
  RR_thigh/1 -> Joint Angles/5, Vector Concatenate/5
  RL_thigh/1 -> Vector Concatenate/6, Joint Angles/6
  FR_thigh/1 -> Vector Concatenate/7, Joint Angles/7
  FL_thigh/1 -> Joint Angles/8, Vector Concatenate/8
  RR_hip/1 -> Joint Angles/9, Vector Concatenate/9
  RL_hip/1 -> Joint Angles/10, Vector Concatenate/10
  FR_hip/1 -> Joint Angles/11, Vector Concatenate/11
  FL_hip/1 -> Joint Angles/12, Vector Concatenate/12
  Vector Concatenate/1 -> joint vector/1

== system unitree_a1_bounding/q_dot ==
  RR_calf : Inport
  RL_calf : Inport  Port=2
  FR_calf : Inport  Port=3
  FL_calf : Inport  Port=4
  RR_thigh : Inport  Port=5
  RL_thigh : Inport  Port=6
  FR_thigh : Inport  Port=7
  FL_thigh : Inport  Port=8
  RR_hip : Inport  Port=9
  RL_hip : Inport  Port=10
  FR_hip : Inport  Port=11
  FL_hip : Inport  Port=12
  Scope : Scope  NumInputPorts=12
  Vector Concatenate : Concatenate  NumInputs=12
  joint vector : Outport
  wires:
  Vector Concatenate/1 -> joint vector/1
  FR_thigh/1 -> Scope/7, Vector Concatenate/7
  FL_hip/1 -> Scope/12, Vector Concatenate/12
  FL_calf/1 -> Scope/4, Vector Concatenate/4
  FL_thigh/1 -> Scope/8, Vector Concatenate/8
  FR_hip/1 -> Scope/11, Vector Concatenate/11
  RR_calf/1 -> Scope/1, Vector Concatenate/1
  RL_hip/1 -> Scope/10, Vector Concatenate/10
  FR_calf/1 -> Scope/3, Vector Concatenate/3
  RR_thigh/1 -> Scope/5, Vector Concatenate/5
  RL_calf/1 -> Scope/2, Vector Concatenate/2
  RL_thigh/1 -> Scope/6, Vector Concatenate/6
  RR_hip/1 -> Scope/9, Vector Concatenate/9

== system unitree_a1_bounding/qd ==
  RR_calf : Inport
  RL_calf : Inport  Port=2
  FR_calf : Inport  Port=3
  FL_calf : Inport  Port=4
  RR_thigh : Inport  Port=5
  RL_thigh : Inport  Port=6
  FR_thigh : Inport  Port=7
  FL_thigh : Inport  Port=8
  RR_hip : Inport  Port=9
  RL_hip : Inport  Port=10
  FR_hip : Inport  Port=11
  FL_hip : Inport  Port=12
  Vector Concatenate : Concatenate  NumInputs=12
  Joint vector : Outport
  wires:
  Vector Concatenate/1 -> Joint vector/1
  FR_hip/1 -> Vector Concatenate/11
  RL_calf/1 -> Vector Concatenate/2
  FL_calf/1 -> Vector Concatenate/4
  RL_thigh/1 -> Vector Concatenate/6
  FL_thigh/1 -> Vector Concatenate/8
  RR_calf/1 -> Vector Concatenate/1
  RR_hip/1 -> Vector Concatenate/9
  FR_calf/1 -> Vector Concatenate/3
  RR_thigh/1 -> Vector Concatenate/5
  FL_hip/1 -> Vector Concatenate/12
  RL_hip/1 -> Vector Concatenate/10
  FR_thigh/1 -> Vector Concatenate/7

== system unitree_a1_bounding/tau ==
  RR_calf : Inport
  RL_calf : Inport  Port=2
  FR_calf : Inport  Port=3
  FL_calf : Inport  Port=4
  RR_thigh : Inport  Port=5
  RL_thigh : Inport  Port=6
  FR_thigh : Inport  Port=7
  FL_thigh : Inport  Port=8
  RR_hip : Inport  Port=9
  RL_hip : Inport  Port=10
  FR_hip : Inport  Port=11
  FL_hip : Inport  Port=12
  Joint Torques : Scope  NumInputPorts=12
  Vector Concatenate : Concatenate  NumInputs=12
  joint vector : Outport
  wires:
  Vector Concatenate/1 -> joint vector/1
  FR_thigh/1 -> Joint Torques/7, Vector Concatenate/7
  FL_hip/1 -> Joint Torques/12, Vector Concatenate/12
  FL_calf/1 -> Joint Torques/4, Vector Concatenate/4
  FL_thigh/1 -> Joint Torques/8, Vector Concatenate/8
  FR_hip/1 -> Joint Torques/11, Vector Concatenate/11
  RR_calf/1 -> Joint Torques/1, Vector Concatenate/1
  RL_hip/1 -> Joint Torques/10, Vector Concatenate/10
  FR_calf/1 -> Joint Torques/3, Vector Concatenate/3
  RR_thigh/1 -> Joint Torques/5, Vector Concatenate/5
  RL_calf/1 -> Joint Torques/2, Vector Concatenate/2
  RL_thigh/1 -> Joint Torques/6, Vector Concatenate/6
  RR_hip/1 -> Joint Torques/9, Vector Concatenate/9

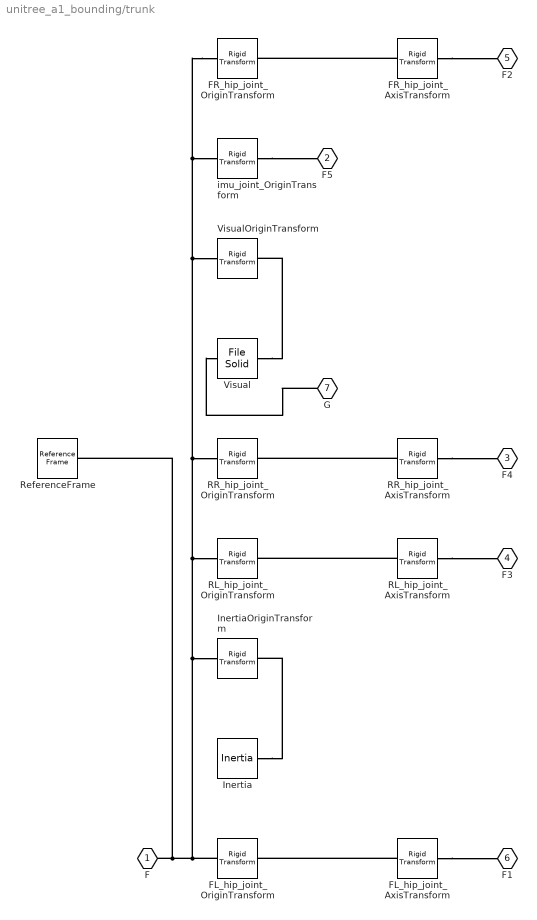
== system unitree_a1_bounding/trunk ==
  FL_hip_joint_AxisTransform : sm_lib/Frames and Transforms/Rigid Transform  TranslationMethod=Cartesian  TranslationStandardOffset=0  TranslationLengthUnit=m  TranslationStandardAxis=+Z  TranslationCartesianOffset=[0, 0, 0]  TranslationROffset=0  TranslationROffsetUnits=m  TranslationZOffset=0  TranslationZOffsetUnits=m  TranslationThetaOffset=0  TranslationThetaOffsetUnits=deg  RotationMethod=ArbitraryAxis  RotationAngleUnits=rad  RotationStandardAxis=+Z  RotationAngle=1.570796326794897  RotationArbitraryAxis=[-0, 1, 0]  FollAlignAxisA=+X  BaseAlignAxisA=+Y  FollAlignAxisB=+Y  BaseAlignAxisB=+Z  RotationSequenceAxes=FollowerAxes  RotationSequence=XYX  RotationSequenceAngles=[0 0 0]  RotationSequenceAnglesUnits=deg  RotationMatrix=[1 0 0; 0 1 0; 0 0 1]  Quaternion=[1 0 0 0]
  FL_hip_joint_OriginTransform : sm_lib/Frames and Transforms/Rigid Transform  TranslationMethod=Cartesian  TranslationStandardOffset=0  TranslationLengthUnit=m  TranslationStandardAxis=+Z  TranslationCartesianOffset=[0.1805, 0.047, 0]  TranslationROffset=0  TranslationROffsetUnits=m  TranslationZOffset=0  TranslationZOffsetUnits=m  TranslationThetaOffset=0  TranslationThetaOffsetUnits=deg  RotationMethod=RotationSequence  RotationAngleUnits=deg  RotationStandardAxis=+Z  RotationAngle=0.0  RotationArbitraryAxis=[0 0 1]  FollAlignAxisA=+X  BaseAlignAxisA=+Y  FollAlignAxisB=+Y  BaseAlignAxisB=+Z  RotationSequenceAxes=BaseAxes  RotationSequence=XYZ  RotationSequenceAngles=[0, 0, 0]  RotationSequenceAnglesUnits=rad  RotationMatrix=[1 0 0; 0 1 0; 0 0 1]  Quaternion=[1 0 0 0]
  FR_hip_joint_AxisTransform : sm_lib/Frames and Transforms/Rigid Transform  TranslationMethod=Cartesian  TranslationStandardOffset=0  TranslationLengthUnit=m  TranslationStandardAxis=+Z  TranslationCartesianOffset=[0, 0, 0]  TranslationROffset=0  TranslationROffsetUnits=m  TranslationZOffset=0  TranslationZOffsetUnits=m  TranslationThetaOffset=0  TranslationThetaOffsetUnits=deg  RotationMethod=ArbitraryAxis  RotationAngleUnits=rad  RotationStandardAxis=+Z  RotationAngle=1.570796326794897  RotationArbitraryAxis=[-0, 1, 0]  FollAlignAxisA=+X  BaseAlignAxisA=+Y  FollAlignAxisB=+Y  BaseAlignAxisB=+Z  RotationSequenceAxes=FollowerAxes  RotationSequence=XYX  RotationSequenceAngles=[0 0 0]  RotationSequenceAnglesUnits=deg  RotationMatrix=[1 0 0; 0 1 0; 0 0 1]  Quaternion=[1 0 0 0]
  FR_hip_joint_OriginTransform : sm_lib/Frames and Transforms/Rigid Transform  TranslationMethod=Cartesian  TranslationStandardOffset=0  TranslationLengthUnit=m  TranslationStandardAxis=+Z  TranslationCartesianOffset=[0.1805, -0.047, 0]  TranslationROffset=0  TranslationROffsetUnits=m  TranslationZOffset=0  TranslationZOffsetUnits=m  TranslationThetaOffset=0  TranslationThetaOffsetUnits=deg  RotationMethod=RotationSequence  RotationAngleUnits=deg  RotationStandardAxis=+Z  RotationAngle=0.0  RotationArbitraryAxis=[0 0 1]  FollAlignAxisA=+X  BaseAlignAxisA=+Y  FollAlignAxisB=+Y  BaseAlignAxisB=+Z  RotationSequenceAxes=BaseAxes  RotationSequence=XYZ  RotationSequenceAngles=[0, 0, 0]  RotationSequenceAnglesUnits=rad  RotationMatrix=[1 0 0; 0 1 0; 0 0 1]  Quaternion=[1 0 0 0]
  Inertia : sm_lib/Body Elements/Inertia  InertiaType=Custom  Mass=6  MassUnits=kg  CenterOfMass=[0, 0, 0]  CenterOfMassUnits=m  MomentsOfInertia=[0.0158533, 0.0377999, 0.0456542]  MomentsOfInertiaUnits=kg*m^2  ProductsOfInertia=[-2.75e-05, -6.109999999999999e-05, -3.66e-05]  ProductsOfInertiaUnits=kg*m^2  GraphicType=None  MarkerShape=Inertia  MarkerSize=20  GraphicVisPropType=SimpleVisualProperties  GraphicDiffuseColor=[0.5 0.5 0.5]  GraphicSpecularColor=[0.5 0.5 0.5 1.0]  GraphicAmbientColor=[0.15 0.15 0.15 1.0]  GraphicEmissiveColor=[0.0 0.0 0.0 1.0]  GraphicShininess=75  GraphicOpacity=1.0
  InertiaOriginTransform : sm_lib/Frames and Transforms/Rigid Transform  TranslationMethod=Cartesian  TranslationStandardOffset=0  TranslationLengthUnit=m  TranslationStandardAxis=+Z  TranslationCartesianOffset=[0, 0.0041, -0.0005]  TranslationROffset=0  TranslationROffsetUnits=m  TranslationZOffset=0  TranslationZOffsetUnits=m  TranslationThetaOffset=0  TranslationThetaOffsetUnits=deg  RotationMethod=RotationSequence  RotationAngleUnits=deg  RotationStandardAxis=+Z  RotationAngle=0.0  RotationArbitraryAxis=[0 0 1]  FollAlignAxisA=+X  BaseAlignAxisA=+Y  FollAlignAxisB=+Y  BaseAlignAxisB=+Z  RotationSequenceAxes=BaseAxes  RotationSequence=XYZ  RotationSequenceAngles=[0, 0, 0]  RotationSequenceAnglesUnits=rad  RotationMatrix=[1 0 0; 0 1 0; 0 0 1]  Quaternion=[1 0 0 0]
  RL_hip_joint_AxisTransform : sm_lib/Frames and Transforms/Rigid Transform  TranslationMethod=Cartesian  TranslationStandardOffset=0  TranslationLengthUnit=m  TranslationStandardAxis=+Z  TranslationCartesianOffset=[0, 0, 0]  TranslationROffset=0  TranslationROffsetUnits=m  TranslationZOffset=0  TranslationZOffsetUnits=m  TranslationThetaOffset=0  TranslationThetaOffsetUnits=deg  RotationMethod=ArbitraryAxis  RotationAngleUnits=rad  RotationStandardAxis=+Z  RotationAngle=1.570796326794897  RotationArbitraryAxis=[-0, 1, 0]  FollAlignAxisA=+X  BaseAlignAxisA=+Y  FollAlignAxisB=+Y  BaseAlignAxisB=+Z  RotationSequenceAxes=FollowerAxes  RotationSequence=XYX  RotationSequenceAngles=[0 0 0]  RotationSequenceAnglesUnits=deg  RotationMatrix=[1 0 0; 0 1 0; 0 0 1]  Quaternion=[1 0 0 0]
  RL_hip_joint_OriginTransform : sm_lib/Frames and Transforms/Rigid Transform  TranslationMethod=Cartesian  TranslationStandardOffset=0  TranslationLengthUnit=m  TranslationStandardAxis=+Z  TranslationCartesianOffset=[-0.1805, 0.047, 0]  TranslationROffset=0  TranslationROffsetUnits=m  TranslationZOffset=0  TranslationZOffsetUnits=m  TranslationThetaOffset=0  TranslationThetaOffsetUnits=deg  RotationMethod=RotationSequence  RotationAngleUnits=deg  RotationStandardAxis=+Z  RotationAngle=0.0  RotationArbitraryAxis=[0 0 1]  FollAlignAxisA=+X  BaseAlignAxisA=+Y  FollAlignAxisB=+Y  BaseAlignAxisB=+Z  RotationSequenceAxes=BaseAxes  RotationSequence=XYZ  RotationSequenceAngles=[0, 0, 0]  RotationSequenceAnglesUnits=rad  RotationMatrix=[1 0 0; 0 1 0; 0 0 1]  Quaternion=[1 0 0 0]
  RR_hip_joint_AxisTransform : sm_lib/Frames and Transforms/Rigid Transform  TranslationMethod=Cartesian  TranslationStandardOffset=0  TranslationLengthUnit=m  TranslationStandardAxis=+Z  TranslationCartesianOffset=[0, 0, 0]  TranslationROffset=0  TranslationROffsetUnits=m  TranslationZOffset=0  TranslationZOffsetUnits=m  TranslationThetaOffset=0  TranslationThetaOffsetUnits=deg  RotationMethod=ArbitraryAxis  RotationAngleUnits=rad  RotationStandardAxis=+Z  RotationAngle=1.570796326794897  RotationArbitraryAxis=[-0, 1, 0]  FollAlignAxisA=+X  BaseAlignAxisA=+Y  FollAlignAxisB=+Y  BaseAlignAxisB=+Z  RotationSequenceAxes=FollowerAxes  RotationSequence=XYX  RotationSequenceAngles=[0 0 0]  RotationSequenceAnglesUnits=deg  RotationMatrix=[1 0 0; 0 1 0; 0 0 1]  Quaternion=[1 0 0 0]
  RR_hip_joint_OriginTransform : sm_lib/Frames and Transforms/Rigid Transform  TranslationMethod=Cartesian  TranslationStandardOffset=0  TranslationLengthUnit=m  TranslationStandardAxis=+Z  TranslationCartesianOffset=[-0.1805, -0.047, 0]  TranslationROffset=0  TranslationROffsetUnits=m  TranslationZOffset=0  TranslationZOffsetUnits=m  TranslationThetaOffset=0  TranslationThetaOffsetUnits=deg  RotationMethod=RotationSequence  RotationAngleUnits=deg  RotationStandardAxis=+Z  RotationAngle=0.0  RotationArbitraryAxis=[0 0 1]  FollAlignAxisA=+X  BaseAlignAxisA=+Y  FollAlignAxisB=+Y  BaseAlignAxisB=+Z  RotationSequenceAxes=BaseAxes  RotationSequence=XYZ  RotationSequenceAngles=[0, 0, 0]  RotationSequenceAnglesUnits=rad  RotationMatrix=[1 0 0; 0 1 0; 0 0 1]  Quaternion=[1 0 0 0]
  ReferenceFrame : sm_lib/Frames and Transforms/Reference Frame
  Visual : sm_lib/Body Elements/File Solid  ExtGeomFileName=meshes/trunk.stl  UnitType=Custom  ExtGeomFileUnits=m  StepReaderType=HEX  ExportConvexHullGeometry=on  InertiaType=Custom  Mass=0  MassUnits=kg  CenterOfMass=[0, 0, 0]  CenterOfMassUnits=m  MomentsOfInertia=[0, 0, 0]  MomentsOfInertiaUnits=kg*m^2  ProductsOfInertia=[0, 0, 0]  ProductsOfInertiaUnits=kg*m^2  BasedOnType=DensityFromFile  Density=1000  DensityUnits=kg/m^3  DoExposeReferenceFrame=on  SerializedFrames=<Frames/>  GraphicType=FromGeometry  MarkerShape=Sphere  MarkerSize=10  GraphicVisPropType=SimpleVisualProperties  GraphicDiffuseColor=[0.8 1.0 1.0]  GraphicSpecularColor=[0.5 0.5 0.5 1.0]  GraphicAmbientColor=[0.15 0.15 0.15 1.0]  GraphicEmissiveColor=[0.0 0.0 0.0 1.0]  GraphicShininess=75  GraphicOpacity=1
  VisualOriginTransform : sm_lib/Frames and Transforms/Rigid Transform  TranslationMethod=Cartesian  TranslationStandardOffset=0  TranslationLengthUnit=m  TranslationStandardAxis=+Z  TranslationCartesianOffset=[0, 0, 0]  TranslationROffset=0  TranslationROffsetUnits=m  TranslationZOffset=0  TranslationZOffsetUnits=m  TranslationThetaOffset=0  TranslationThetaOffsetUnits=deg  RotationMethod=RotationSequence  RotationAngleUnits=deg  RotationStandardAxis=+Z  RotationAngle=0.0  RotationArbitraryAxis=[0 0 1]  FollAlignAxisA=+X  BaseAlignAxisA=+Y  FollAlignAxisB=+Y  BaseAlignAxisB=+Z  RotationSequenceAxes=BaseAxes  RotationSequence=XYZ  RotationSequenceAngles=[0, 0, 0]  RotationSequenceAnglesUnits=rad  RotationMatrix=[1 0 0; 0 1 0; 0 0 1]  Quaternion=[1 0 0 0]
  imu_joint_OriginTransform : sm_lib/Frames and Transforms/Rigid Transform  TranslationMethod=Cartesian  TranslationStandardOffset=0  TranslationLengthUnit=m  TranslationStandardAxis=+Z  TranslationCartesianOffset=[0, 0, 0]  TranslationROffset=0  TranslationROffsetUnits=m  TranslationZOffset=0  TranslationZOffsetUnits=m  TranslationThetaOffset=0  TranslationThetaOffsetUnits=deg  RotationMethod=RotationSequence  RotationAngleUnits=deg  RotationStandardAxis=+Z  RotationAngle=0.0  RotationArbitraryAxis=[0 0 1]  FollAlignAxisA=+X  BaseAlignAxisA=+Y  FollAlignAxisB=+Y  BaseAlignAxisB=+Z  RotationSequenceAxes=BaseAxes  RotationSequence=XYZ  RotationSequenceAngles=[0, 0, 0]  RotationSequenceAnglesUnits=rad  RotationMatrix=[1 0 0; 0 1 0; 0 0 1]  Quaternion=[1 0 0 0]
  F : PMIOPort  Side=Left
  F5 : PMIOPort  Port=2  Side=Right
  F4 : PMIOPort  Port=3  Side=Right
  F3 : PMIOPort  Port=4  Side=Right
  F2 : PMIOPort  Port=5  Side=Right
  F1 : PMIOPort  Port=6  Side=Right
  G : PMIOPort  Port=7  Side=Right
  connections:
  FL_hip_joint_AxisTransform/RConn1 -- F1/RConn1
  FL_hip_joint_AxisTransform/LConn1 -- FL_hip_joint_OriginTransform/RConn1
  FR_hip_joint_AxisTransform/RConn1 -- F2/RConn1
  FR_hip_joint_AxisTransform/LConn1 -- FR_hip_joint_OriginTransform/RConn1
  Inertia/RConn1 -- InertiaOriginTransform/RConn1
  RL_hip_joint_AxisTransform/RConn1 -- F3/RConn1
  RL_hip_joint_AxisTransform/LConn1 -- RL_hip_joint_OriginTransform/RConn1
  RR_hip_joint_AxisTransform/RConn1 -- F4/RConn1
  RR_hip_joint_AxisTransform/LConn1 -- RR_hip_joint_OriginTransform/RConn1
  FR_hip_joint_OriginTransform/LConn1 -- FL_hip_joint_OriginTransform/LConn1 -- ReferenceFrame/RConn1 -- F/RConn1 -- InertiaOriginTransform/LConn1 -- RL_hip_joint_OriginTransform/LConn1 -- RR_hip_joint_OriginTransform/LConn1 -- VisualOriginTransform/LConn1 -- imu_joint_OriginTransform/LConn1
  Visual/RConn1 -- VisualOriginTransform/RConn1
  imu_joint_OriginTransform/RConn1 -- F5/RConn1
  G/RConn1 -- Visual/LConn1

== system unitree_a1_bounding/vd_COM ==
  Constant3 : Constant  Value=0
  Ramp : simulink/Sources/Ramp  slope=0.2  start=1.95  InitialOutput=0.1
  Saturation1 : Saturate  UpperLimit=0.6  LowerLimit=-0.6
  Vector Concatenate3 : Concatenate  NumInputs=3
  Out1 : Outport
  wires:
  Constant3/1 -> Vector Concatenate3/2, Vector Concatenate3/3
  Vector Concatenate3/1 -> Out1/1
  Ramp/1 -> Saturation1/1
  Saturation1/1 -> Vector Concatenate3/1

== system unitree_a1_bounding/wd_COM ==
  Constant3 : Constant  Value=0
  Ramp : simulink/Sources/Ramp  slope=0.2  start=1.95  InitialOutput=0.1
  Saturation1 : Saturate  UpperLimit=0.6  LowerLimit=-0.6
  Vector Concatenate3 : Concatenate  NumInputs=3
  w : Outport
  wires:
  Constant3/1 -> Vector Concatenate3/2, Vector Concatenate3/1
  Vector Concatenate3/1 -> w/1
  Ramp/1 -> Saturation1/1
  Saturation1/1 -> Vector Concatenate3/3
